simulink model "pi_hooke"  (R2019a)
settings: Solver=VariableStepAuto  StartTime=0.0  StopTime=10  RelTol=1e-3
values from neighbouring files (symbols this model uses):
  den = double(den)    [main.m]
  Ki = x2    [cost.m]
  Kp = x1    [cost.m]
  num = double(num)    [main.m]
settings Model: Creator=Furka  LastModifiedBy=Furka

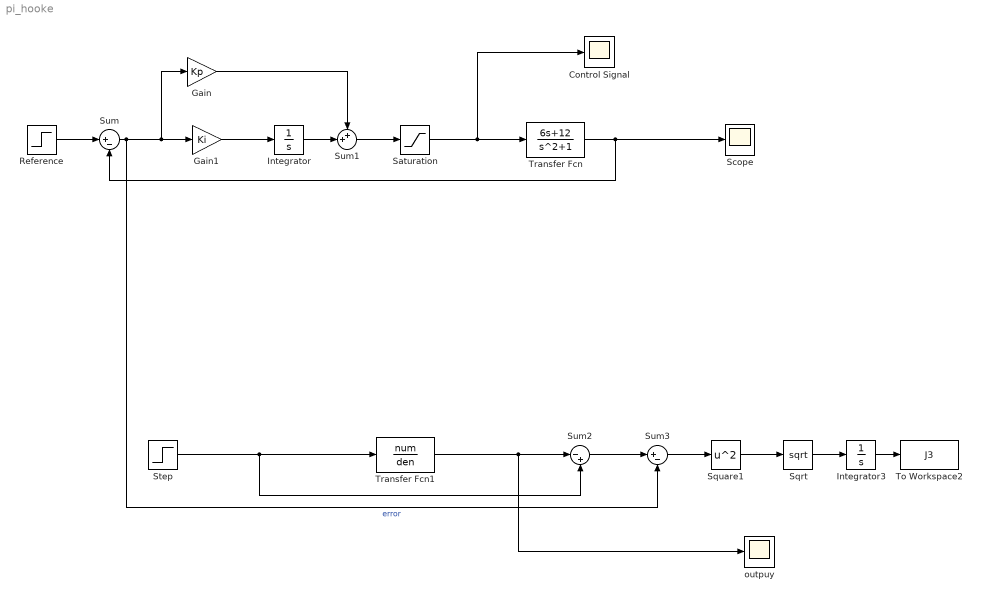
== system pi_hooke ==
  Control Signal : Scope
  Gain : Gain  Gain=Kp
  Gain1 : Gain  Gain=Ki
  Integrator : Integrator
  Integrator3 : Integrator
  Reference : Step  Time=0  SampleTime=0
  Saturation : Saturate  UpperLimit=35  LowerLimit=-1
  Scope : Scope
  Sqrt : Sqrt  SaturateOnIntegerOverflow=on
  Square1 : Math  Operator=square  SaturateOnIntegerOverflow=on
  Step : Step  Time=0  SampleTime=0
  Sum : Sum  Inputs=|+-
  Sum1 : Sum  Inputs=++|
  Sum2 : Sum  Inputs=|-+
  Sum3 : Sum  Inputs=|+-
  To Workspace2 : ToWorkspace  VariableName=J3  SampleTime=-1
  Transfer Fcn : TransferFcn  Numerator=[6 12]  Denominator=[1 0 1]
  Transfer Fcn1 : TransferFcn  Numerator=num  Denominator=den
  "outpuy " : Scope
  wires:
  Reference/1 -> Sum/1
  Gain1/1 -> Integrator/1
  Integrator/1 -> Sum1/2
  Gain/1 -> Sum1/1
  Sum/1 -> Sum3/2, Gain/1, Gain1/1  "error"
  Transfer Fcn/1 -> Sum/2, Scope/1
  Sum2/1 -> Sum3/1
  Sum3/1 -> Square1/1
  Square1/1 -> Sqrt/1
  Sqrt/1 -> Integrator3/1
  Integrator3/1 -> To Workspace2/1
  Transfer Fcn1/1 -> "outpuy "/1, Sum2/1
  Step/1 -> Transfer Fcn1/1, Sum2/2
  Sum1/1 -> Saturation/1
  Saturation/1 -> Control Signal/1, Transfer Fcn/1
